simulink model "figure_2_5"  (R2026a)
settings: Solver=ode5  FixedStep=1e-4
settings Model: Creator=yagmu  LastModifiedBy=yagmu

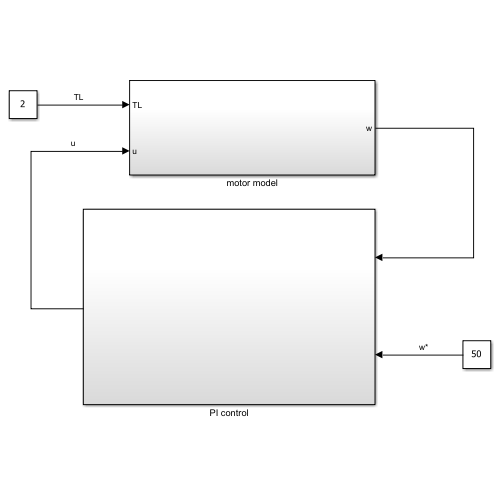
[thumbnail: Simulink's stored preview of the top-level diagram]
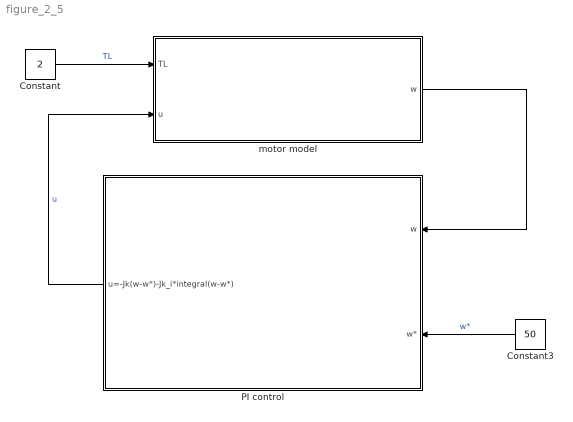
== system figure_2_5 ==
  Constant : Constant  Value=2
  Constant3 : Constant  Value=50
  PI control : Subsystem
      settings: PortSchema="{\"entries\":[{\"content\":{\"sides\":[{\"content\":{\"connectorIds\":[\"Out1\"]},\"type\":\"ConnectorPlacement.EquallySpacedRectSide\",\"uuid\":\"710ac4ad-407c-4c0a-912c-3424909594c3\"},{\"content\":{\"connectorIds\":[\"In1\",\"In2\"],\"side\":\"RIGHT\"},\"type\":\"ConnectorPlacement.EquallySpacedRectSide\",\"uuid\":\"58c339e6-c64a-40ec-a9ea-97bd3e4c8664\"},{\"content\":{\"side\":\"TOP\"},\"type\":\"ConnectorPlacement.EquallySpacedRectSide\",\"uuid\":\"1ba305bc-8c3f-41cb-bb55-94fbe652244d\"}]},\"type\":\"ConnectorPlacement.EquallySpacedConnector\",\"uuid\":\"41553efe-4509-43cb-bfc1-ed5b56513470\"}],\"packageUris\":[\"http://schema.mathworks.com/mf0/Connector/R2020b\"],\"version\":\"1.0\"}"
  motor model : Subsystem
  wires:
  Constant3/1 -> PI control/2(w*)  "w*"
  Constant/1 -> motor model/1(TL)  "TL"
  PI control/1(u=-Jk(w-w*)-Jk_i*integral(w-w*)) -> motor model/2(u)  "u"
  motor model/1(w) -> PI control/1(w)

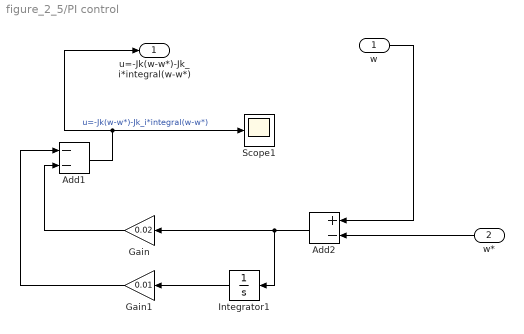
== system figure_2_5/PI control ==
  w : Inport
  w* : Inport  Port=2
  Add1 : Sum  Inputs=--
  Add2 : Sum  Inputs=+-
  Gain : Gain  Gain=0.02
  Gain1 : Gain  Gain=0.01
  Integrator1 : Integrator
  Scope1 : Scope
      settings: ActiveDisplayYMinimum=1.8875000000000441  ActiveDisplayYMaximum=2.0124999999996005
  u=-Jk(w-w*)-Jk_i*integral(w-w*) : Outport
  wires:
  Gain/1 -> Add1/2
  w*/1 -> Add2/2
  Integrator1/1 -> Gain1/1
  Add1/1 -> u=-Jk(w-w*)-Jk_i*integral(w-w*)/1, Scope1/1  "u=-Jk(w-w*)-Jk_i*integral(w-w*)"
  Gain1/1 -> Add1/1
  Add2/1 -> Integrator1/1, Gain/1
  w/1 -> Add2/1

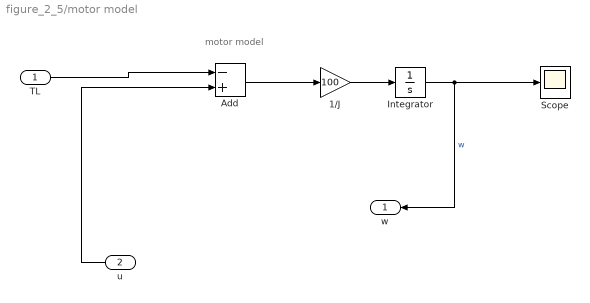
== system figure_2_5/motor model ==
  note: motor model
  TL : Inport
  u : Inport  Port=2
  1/J : Gain  Gain=100
  Add : Sum  Inputs=-+
  Integrator : Integrator  InitialCondition=50
  Scope : Scope
      settings: ActiveDisplayYMinimum=-32.772874263574465  ActiveDisplayYMaximum=59.196986029286052
  w : Outport
  wires:
  Integrator/1 -> w/1, Scope/1  "w"
  Add/1 -> 1/J/1
  1/J/1 -> Integrator/1
  u/1 -> Add/2
  TL/1 -> Add/1
